simulink model "secondOrderComparison"  (R2020b)
settings: Solver=VariableStepAuto  StartTime=0.0  StopTime=10.0  RelTol=1e-3
libraries: simulink x3
settings Model: Creator=jaagt  LastModifiedBy=jaagt

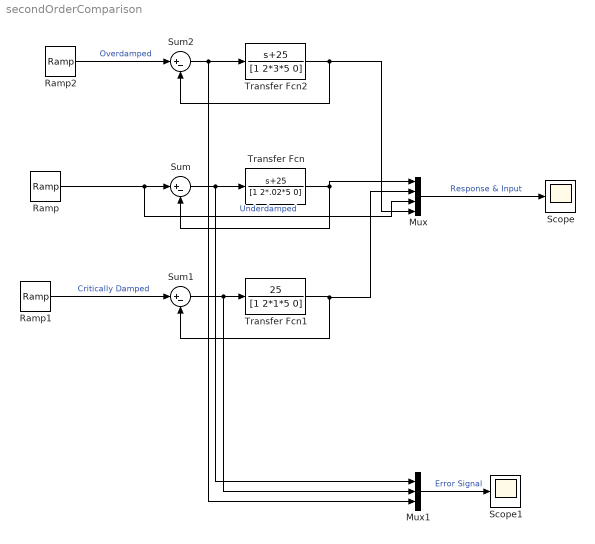
== system secondOrderComparison ==
  Mux : Mux
  Mux1 : Mux  Inputs=3
  Ramp : simulink/Sources/Ramp  slope=1  start=0  InitialOutput=0
  Ramp1 : simulink/Sources/Ramp  slope=1  start=0  InitialOutput=0
  Ramp2 : simulink/Sources/Ramp  slope=1  start=0  InitialOutput=0
  Scope : Scope
  Scope1 : Scope
  Sum : Sum  Inputs=|+-
  Sum1 : Sum  Inputs=|+-
  Sum2 : Sum  Inputs=|+-
  Transfer Fcn : TransferFcn  Numerator=[0 1 25]  Denominator=[1 2*.02*5 0]
  Transfer Fcn1 : TransferFcn  Numerator=[0 0 25]  Denominator=[1 2*1*5 0]
  Transfer Fcn2 : TransferFcn  Numerator=[0 1 25]  Denominator=[1 2*3*5 0]
  wires:
  Ramp/1 -> Mux/3, Sum/1  "Underdamped"
  Sum/1 -> Mux1/1, Transfer Fcn/1
  Transfer Fcn/1 -> Mux/1, Sum/2
  Sum1/1 -> Mux1/2, Transfer Fcn1/1
  Transfer Fcn1/1 -> Mux/2, Sum1/2
  Ramp1/1 -> Sum1/1  "Critically Damped"
  Mux/1 -> Scope/1  "Response & Input"
  Mux1/1 -> Scope1/1  "Error Signal"
  Sum2/1 -> Mux1/3, Transfer Fcn2/1
  Transfer Fcn2/1 -> Mux/4, Sum2/2
  Ramp2/1 -> Sum2/1  "Overdamped"
